simulink model "Feeder_1"  (Simulink 8.8)
settings: Solver=ode4  StartTime=0.0  StopTime=inf  FixedStep=Ts  RelTol=1e-3  EnableMultiTasking=on
PreLoadFcn:
  | Ts=125e-6;Core_Num = 0; np=1; nq=1; Vmin=.9;
PostLoadFcn:
  | Ts=125e-6;Core_Num = 0; np=1; nq=1; Vmin=.9;
InitFcn:
  | Ts=125e-6;Core_Num = 0; np=1; nq=1; Vmin=.9;
undefined symbols (not defined in the file or in its folder): another_event_name, DiscIntNeverNeededParam, I, j, Left, my_event_name, Right, type, V, X
libraries: powerlib x316, powerlib_meascontrol x227, simulink_extras x78, simulink x25, rtio_generic_c37_118 x22, ssn_lib x9, rtlab x6, powerlib_extras x3, artemis x1, rtio_opalrt_ml605ex1 x1, rtio_spectracom x1, rtio_generic_ethernet x1
(part 5 of 14)

== system Feeder_1/SS_PMU/Subsystem35 ==
  PMU in : Inport
  Bus Selector : BusSelector  OutputSignals=Measurements,FREQ,FROC
  Constant28 : Constant  Value=-1
  Constant29 : Constant  Value=-1
  Subsystem : Subsystem
  Phasors : Outport
  Analog : Outport  Port=2
  Ditigal : Outport  Port=3
  FREQ : Outport  Port=4
  FROC : Outport  Port=5
  wires:
  Subsystem/1(Out1) -> Bus Selector/1
  Bus Selector/1 -> Phasors/1  "<Measurements>"
  PMU in/1 -> Subsystem/1(In1)
  Constant28/1 -> Analog/1
  Constant29/1 -> Ditigal/1
  Bus Selector/2 -> FREQ/1  "<FREQ>"
  Bus Selector/3 -> FROC/1  "<FROC>"

== system Feeder_1/SS_PMU/Subsystem36 ==
  PMU in : Inport
  Bus Selector : BusSelector  OutputSignals=Measurements,FREQ,FROC
  Constant28 : Constant  Value=-1
  Constant29 : Constant  Value=-1
  Subsystem : Subsystem
  Phasors : Outport
  Analog : Outport  Port=2
  Ditigal : Outport  Port=3
  FREQ : Outport  Port=4
  FROC : Outport  Port=5
  wires:
  Subsystem/1(Out1) -> Bus Selector/1
  Bus Selector/1 -> Phasors/1  "<Measurements>"
  PMU in/1 -> Subsystem/1(In1)
  Constant28/1 -> Analog/1
  Constant29/1 -> Ditigal/1
  Bus Selector/2 -> FREQ/1  "<FREQ>"
  Bus Selector/3 -> FROC/1  "<FROC>"

== system Feeder_1/SS_PMU/Subsystem37 ==
  PMU in : Inport
  Bus Selector : BusSelector  OutputSignals=Measurements,FREQ,FROC
  Constant28 : Constant  Value=-1
  Constant29 : Constant  Value=-1
  Subsystem : Subsystem
  Phasors : Outport
  Analog : Outport  Port=2
  Ditigal : Outport  Port=3
  FREQ : Outport  Port=4
  FROC : Outport  Port=5
  wires:
  Subsystem/1(Out1) -> Bus Selector/1
  Bus Selector/1 -> Phasors/1  "<Measurements>"
  PMU in/1 -> Subsystem/1(In1)
  Constant28/1 -> Analog/1
  Constant29/1 -> Ditigal/1
  Bus Selector/2 -> FREQ/1  "<FREQ>"
  Bus Selector/3 -> FROC/1  "<FROC>"

== system Feeder_1/SS_PMU/Subsystem38 ==
  PMU in : Inport
  Bus Selector : BusSelector  OutputSignals=Measurements,FREQ,FROC
  Constant28 : Constant  Value=-1
  Constant29 : Constant  Value=-1
  Subsystem : Subsystem
  Phasors : Outport
  Analog : Outport  Port=2
  Ditigal : Outport  Port=3
  FREQ : Outport  Port=4
  FROC : Outport  Port=5
  wires:
  Subsystem/1(Out1) -> Bus Selector/1
  Bus Selector/1 -> Phasors/1  "<Measurements>"
  PMU in/1 -> Subsystem/1(In1)
  Constant28/1 -> Analog/1
  Constant29/1 -> Ditigal/1
  Bus Selector/2 -> FREQ/1  "<FREQ>"
  Bus Selector/3 -> FROC/1  "<FROC>"

== system Feeder_1/SS_PMU/Subsystem39 ==
  PMU in : Inport
  Bus Selector : BusSelector  OutputSignals=Measurements,FREQ,FROC
  Constant28 : Constant  Value=-1
  Constant29 : Constant  Value=-1
  Subsystem : Subsystem
  Phasors : Outport
  Analog : Outport  Port=2
  Ditigal : Outport  Port=3
  FREQ : Outport  Port=4
  FROC : Outport  Port=5
  wires:
  Subsystem/1(Out1) -> Bus Selector/1
  Bus Selector/1 -> Phasors/1  "<Measurements>"
  PMU in/1 -> Subsystem/1(In1)
  Constant28/1 -> Analog/1
  Constant29/1 -> Ditigal/1
  Bus Selector/2 -> FREQ/1  "<FREQ>"
  Bus Selector/3 -> FROC/1  "<FROC>"

== system Feeder_1/SS_PMU/Subsystem4 ==
  Measurements : Inport
  Demux7 : Demux  Outputs=6
  Demux8 : Demux  Outputs=6
  Mux5 : Mux  Inputs=12
  Subsystem : Subsystem
  Phasors : Outport
  Phasor_Freq : Outport  Port=2
  FROC : Outport  Port=3
  wires:
  Mux5/1 -> Phasors/1
  Demux7/4 -> [Phase_Va]
  Demux7/1 -> [Mag_Va]
  Demux7/2 -> [Mag_Vb]
  Demux7/3 -> [Mag_Vc]
  Subsystem/1(Phasors_Vabc) -> Demux7/1
  Demux7/6 -> [Phase_Vc]
  Demux7/5 -> [Phase_Vb]
  Subsystem/3(Phasor_Freq) -> Phasor_Freq/1
  Measurements/1 -> Subsystem/1(Measurements1)
  Subsystem/4(Phasor_DTFreq) -> FROC/1
  Demux8/2 -> [Mag_Ib]
  Demux8/4 -> [Phase_Ia]
  Demux8/5 -> [Phase_Ib]
  Subsystem/2(Phasors_Iabc) -> Demux8/1
  Demux8/3 -> [Mag_Ic]
  Demux8/1 -> [Mag_Ia]
  Demux8/6 -> [Phase_Ic]
  [Phase_Ic] -> Mux5/12
  [Mag_Ic] -> Mux5/11
  [Phase_Ib] -> Mux5/10
  [Mag_Ib] -> Mux5/9
  [Phase_Ia] -> Mux5/8
  [Mag_Ia] -> Mux5/7
  [Phase_Vc] -> Mux5/6
  [Mag_Vc] -> Mux5/5
  [Phase_Vb] -> Mux5/4
  [Mag_Vb] -> Mux5/3
  [Phase_Va] -> Mux5/2
  [Mag_Va] -> Mux5/1

== system Feeder_1/SS_PMU/Subsystem40 ==
  PMU in : Inport
  Bus Selector : BusSelector  OutputSignals=Measurements,FREQ,FROC
  Constant28 : Constant  Value=-1
  Constant29 : Constant  Value=-1
  Subsystem : Subsystem
  Phasors : Outport
  Analog : Outport  Port=2
  Ditigal : Outport  Port=3
  FREQ : Outport  Port=4
  FROC : Outport  Port=5
  wires:
  Subsystem/1(Out1) -> Bus Selector/1
  Bus Selector/1 -> Phasors/1  "<Measurements>"
  PMU in/1 -> Subsystem/1(In1)
  Constant28/1 -> Analog/1
  Constant29/1 -> Ditigal/1
  Bus Selector/2 -> FREQ/1  "<FREQ>"
  Bus Selector/3 -> FROC/1  "<FROC>"

== system Feeder_1/SS_PMU/Subsystem41 ==
  PMU in : Inport
  Bus Selector : BusSelector  OutputSignals=Measurements,FREQ,FROC
  Constant28 : Constant  Value=-1
  Constant29 : Constant  Value=-1
  Subsystem : Subsystem
  Phasors : Outport
  Analog : Outport  Port=2
  Ditigal : Outport  Port=3
  FREQ : Outport  Port=4
  FROC : Outport  Port=5
  wires:
  Subsystem/1(Out1) -> Bus Selector/1
  Bus Selector/1 -> Phasors/1  "<Measurements>"
  PMU in/1 -> Subsystem/1(In1)
  Constant28/1 -> Analog/1
  Constant29/1 -> Ditigal/1
  Bus Selector/2 -> FREQ/1  "<FREQ>"
  Bus Selector/3 -> FROC/1  "<FROC>"

== system Feeder_1/SS_PMU/Subsystem42 ==
  PMU in : Inport
  Bus Selector : BusSelector  OutputSignals=Measurements,FREQ,FROC
  Constant28 : Constant  Value=-1
  Constant29 : Constant  Value=-1
  Subsystem : Subsystem
  Phasors : Outport
  Analog : Outport  Port=2
  Ditigal : Outport  Port=3
  FREQ : Outport  Port=4
  FROC : Outport  Port=5
  wires:
  Subsystem/1(Out1) -> Bus Selector/1
  Bus Selector/1 -> Phasors/1  "<Measurements>"
  PMU in/1 -> Subsystem/1(In1)
  Constant28/1 -> Analog/1
  Constant29/1 -> Ditigal/1
  Bus Selector/2 -> FREQ/1  "<FREQ>"
  Bus Selector/3 -> FROC/1  "<FROC>"

== system Feeder_1/SS_PMU/Subsystem43 ==
  PMU in : Inport
  Bus Selector : BusSelector  OutputSignals=Measurements,FREQ,FROC
  Constant28 : Constant  Value=-1
  Constant29 : Constant  Value=-1
  Subsystem : Subsystem
  Phasors : Outport
  Analog : Outport  Port=2
  Ditigal : Outport  Port=3
  FREQ : Outport  Port=4
  FROC : Outport  Port=5
  wires:
  Subsystem/1(Out1) -> Bus Selector/1
  Bus Selector/1 -> Phasors/1  "<Measurements>"
  PMU in/1 -> Subsystem/1(In1)
  Constant28/1 -> Analog/1
  Constant29/1 -> Ditigal/1
  Bus Selector/2 -> FREQ/1  "<FREQ>"
  Bus Selector/3 -> FROC/1  "<FROC>"

== system Feeder_1/SS_PMU/Subsystem44 ==
  PMU in : Inport
  Bus Selector : BusSelector  OutputSignals=Measurements,FREQ,FROC
  Constant28 : Constant  Value=-1
  Constant29 : Constant  Value=-1
  Subsystem : Subsystem
  Phasors : Outport
  Analog : Outport  Port=2
  Ditigal : Outport  Port=3
  FREQ : Outport  Port=4
  FROC : Outport  Port=5
  wires:
  Subsystem/1(Out1) -> Bus Selector/1
  Bus Selector/1 -> Phasors/1  "<Measurements>"
  PMU in/1 -> Subsystem/1(In1)
  Constant28/1 -> Analog/1
  Constant29/1 -> Ditigal/1
  Bus Selector/2 -> FREQ/1  "<FREQ>"
  Bus Selector/3 -> FROC/1  "<FROC>"

== system Feeder_1/SS_PMU/Subsystem5 ==
  Measurements : Inport
  Demux7 : Demux  Outputs=6
  Demux8 : Demux  Outputs=6
  Mux5 : Mux  Inputs=12
  Subsystem : Subsystem
  Phasors : Outport
  Phasor_Freq : Outport  Port=2
  FROC : Outport  Port=3
  wires:
  Mux5/1 -> Phasors/1
  Demux7/4 -> [Phase_Va]
  Demux7/1 -> [Mag_Va]
  Demux7/2 -> [Mag_Vb]
  Demux7/3 -> [Mag_Vc]
  Subsystem/1(Phasors_Vabc) -> Demux7/1
  Demux7/6 -> [Phase_Vc]
  Demux7/5 -> [Phase_Vb]
  Subsystem/3(Phasor_Freq) -> Phasor_Freq/1
  Measurements/1 -> Subsystem/1(Measurements1)
  Subsystem/4(Phasor_DTFreq) -> FROC/1
  Demux8/2 -> [Mag_Ib]
  Demux8/4 -> [Phase_Ia]
  Demux8/5 -> [Phase_Ib]
  Subsystem/2(Phasors_Iabc) -> Demux8/1
  Demux8/3 -> [Mag_Ic]
  Demux8/1 -> [Mag_Ia]
  Demux8/6 -> [Phase_Ic]
  [Phase_Ic] -> Mux5/12
  [Mag_Ic] -> Mux5/11
  [Phase_Ib] -> Mux5/10
  [Mag_Ib] -> Mux5/9
  [Phase_Ia] -> Mux5/8
  [Mag_Ia] -> Mux5/7
  [Phase_Vc] -> Mux5/6
  [Mag_Vc] -> Mux5/5
  [Phase_Vb] -> Mux5/4
  [Mag_Vb] -> Mux5/3
  [Phase_Va] -> Mux5/2
  [Mag_Va] -> Mux5/1

== system Feeder_1/SS_PMU/Subsystem6 ==
  Measurements : Inport
  Demux7 : Demux  Outputs=6
  Demux8 : Demux  Outputs=6
  Mux5 : Mux  Inputs=12
  Subsystem : Subsystem
  Phasors : Outport
  Phasor_Freq : Outport  Port=2
  FROC : Outport  Port=3
  wires:
  Mux5/1 -> Phasors/1
  Demux7/4 -> [Phase_Va]
  Demux7/1 -> [Mag_Va]
  Demux7/2 -> [Mag_Vb]
  Demux7/3 -> [Mag_Vc]
  Subsystem/1(Phasors_Vabc) -> Demux7/1
  Demux7/6 -> [Phase_Vc]
  Demux7/5 -> [Phase_Vb]
  Subsystem/3(Phasor_Freq) -> Phasor_Freq/1
  Measurements/1 -> Subsystem/1(Measurements1)
  Subsystem/4(Phasor_DTFreq) -> FROC/1
  Demux8/2 -> [Mag_Ib]
  Demux8/4 -> [Phase_Ia]
  Demux8/5 -> [Phase_Ib]
  Subsystem/2(Phasors_Iabc) -> Demux8/1
  Demux8/3 -> [Mag_Ic]
  Demux8/1 -> [Mag_Ia]
  Demux8/6 -> [Phase_Ic]
  [Phase_Ic] -> Mux5/12
  [Mag_Ic] -> Mux5/11
  [Phase_Ib] -> Mux5/10
  [Mag_Ib] -> Mux5/9
  [Phase_Ia] -> Mux5/8
  [Mag_Ia] -> Mux5/7
  [Phase_Vc] -> Mux5/6
  [Mag_Vc] -> Mux5/5
  [Phase_Vb] -> Mux5/4
  [Mag_Vb] -> Mux5/3
  [Phase_Va] -> Mux5/2
  [Mag_Va] -> Mux5/1

== system Feeder_1/SS_PMU/Subsystem7 ==
  Measurements : Inport
  Demux7 : Demux  Outputs=6
  Demux8 : Demux  Outputs=6
  Mux5 : Mux  Inputs=12
  Subsystem : Subsystem
  Phasors : Outport
  Phasor_Freq : Outport  Port=2
  FROC : Outport  Port=3
  wires:
  Mux5/1 -> Phasors/1
  Demux7/4 -> [Phase_Va]
  Demux7/1 -> [Mag_Va]
  Demux7/2 -> [Mag_Vb]
  Demux7/3 -> [Mag_Vc]
  Subsystem/1(Phasors_Vabc) -> Demux7/1
  Demux7/6 -> [Phase_Vc]
  Demux7/5 -> [Phase_Vb]
  Subsystem/3(Phasor_Freq) -> Phasor_Freq/1
  Measurements/1 -> Subsystem/1(Measurements1)
  Subsystem/4(Phasor_DTFreq) -> FROC/1
  Demux8/2 -> [Mag_Ib]
  Demux8/4 -> [Phase_Ia]
  Demux8/5 -> [Phase_Ib]
  Subsystem/2(Phasors_Iabc) -> Demux8/1
  Demux8/3 -> [Mag_Ic]
  Demux8/1 -> [Mag_Ia]
  Demux8/6 -> [Phase_Ic]
  [Phase_Ic] -> Mux5/12
  [Mag_Ic] -> Mux5/11
  [Phase_Ib] -> Mux5/10
  [Mag_Ib] -> Mux5/9
  [Phase_Ia] -> Mux5/8
  [Mag_Ia] -> Mux5/7
  [Phase_Vc] -> Mux5/6
  [Mag_Vc] -> Mux5/5
  [Phase_Vb] -> Mux5/4
  [Mag_Vb] -> Mux5/3
  [Phase_Va] -> Mux5/2
  [Mag_Va] -> Mux5/1

== system Feeder_1/SS_PMU/Subsystem8 ==
  Measurements : Inport
  Demux7 : Demux  Outputs=6
  Demux8 : Demux  Outputs=6
  Mux5 : Mux  Inputs=12
  Subsystem : Subsystem
  Phasors : Outport
  Phasor_Freq : Outport  Port=2
  FROC : Outport  Port=3
  wires:
  Mux5/1 -> Phasors/1
  Demux7/4 -> [Phase_Va]
  Demux7/1 -> [Mag_Va]
  Demux7/2 -> [Mag_Vb]
  Demux7/3 -> [Mag_Vc]
  Subsystem/1(Phasors_Vabc) -> Demux7/1
  Demux7/6 -> [Phase_Vc]
  Demux7/5 -> [Phase_Vb]
  Subsystem/3(Phasor_Freq) -> Phasor_Freq/1
  Measurements/1 -> Subsystem/1(Measurements1)
  Subsystem/4(Phasor_DTFreq) -> FROC/1
  Demux8/2 -> [Mag_Ib]
  Demux8/4 -> [Phase_Ia]
  Demux8/5 -> [Phase_Ib]
  Subsystem/2(Phasors_Iabc) -> Demux8/1
  Demux8/3 -> [Mag_Ic]
  Demux8/1 -> [Mag_Ia]
  Demux8/6 -> [Phase_Ic]
  [Phase_Ic] -> Mux5/12
  [Mag_Ic] -> Mux5/11
  [Phase_Ib] -> Mux5/10
  [Mag_Ib] -> Mux5/9
  [Phase_Ia] -> Mux5/8
  [Mag_Ia] -> Mux5/7
  [Phase_Vc] -> Mux5/6
  [Mag_Vc] -> Mux5/5
  [Phase_Vb] -> Mux5/4
  [Mag_Vb] -> Mux5/3
  [Phase_Va] -> Mux5/2
  [Mag_Va] -> Mux5/1

== system Feeder_1/SS_PMU/Subsystem9 ==
  Measurements : Inport
  Demux7 : Demux  Outputs=6
  Demux8 : Demux  Outputs=6
  Mux5 : Mux  Inputs=12
  Subsystem : Subsystem
  Phasors : Outport
  Phasor_Freq : Outport  Port=2
  FROC : Outport  Port=3
  wires:
  Mux5/1 -> Phasors/1
  Demux7/4 -> [Phase_Va]
  Demux7/1 -> [Mag_Va]
  Demux7/2 -> [Mag_Vb]
  Demux7/3 -> [Mag_Vc]
  Subsystem/1(Phasors_Vabc) -> Demux7/1
  Demux7/6 -> [Phase_Vc]
  Demux7/5 -> [Phase_Vb]
  Subsystem/3(Phasor_Freq) -> Phasor_Freq/1
  Measurements/1 -> Subsystem/1(Measurements1)
  Subsystem/4(Phasor_DTFreq) -> FROC/1
  Demux8/2 -> [Mag_Ib]
  Demux8/4 -> [Phase_Ia]
  Demux8/5 -> [Phase_Ib]
  Subsystem/2(Phasors_Iabc) -> Demux8/1
  Demux8/3 -> [Mag_Ic]
  Demux8/1 -> [Mag_Ia]
  Demux8/6 -> [Phase_Ic]
  [Phase_Ic] -> Mux5/12
  [Mag_Ic] -> Mux5/11
  [Phase_Ib] -> Mux5/10
  [Mag_Ib] -> Mux5/9
  [Phase_Ia] -> Mux5/8
  [Mag_Ia] -> Mux5/7
  [Phase_Vc] -> Mux5/6
  [Mag_Vc] -> Mux5/5
  [Phase_Vb] -> Mux5/4
  [Mag_Vb] -> Mux5/3
  [Phase_Va] -> Mux5/2
  [Mag_Va] -> Mux5/1

== system Feeder_1/SM_NG/Dynamic Load BCDC2/Single-Phase Dynamic Load1 ==
  P : Inport
  Q : Inport  Port=2
  Active : Gain  Gain=900000
  Active1 : Gain  Gain=400000
  Controlled Current Source : powerlib/Electrical Sources/Controlled Current Source  Initialize=on  Source_Type=AC  Amplitude=0  Phase=0  Frequency=0  Measurements=None
  Gain : Gain  Gain=-1
  Mux8 : Mux  Inputs=2
  Voltage Measurement1 : powerlib/Measurements/Voltage Measurement  PhasorSimulation=off  OutputType=Complex  PSBequivalent=0
  model : Subsystem
  a : PMIOPort  Tag=PMCPort  Port=1  Side=Left
  b : PMIOPort  Tag=PMCPort  Port=2  Side=Left
  wires:
  Mux8/1 -> model/2(PQ)
  Voltage Measurement1/1 -> model/1(v)
  model/1(i) -> Gain/1
  Gain/1 -> Controlled Current Source/1
  Active/1 -> Mux8/1
  Active1/1 -> Mux8/2
  P/1 -> Active/1
  Q/1 -> Active1/1
  connections:
  Voltage Measurement1/LConn1 -- a/RConn1 -- Controlled Current Source/RConn1
  Voltage Measurement1/LConn2 -- b/RConn1 -- Controlled Current Source/LConn1

== system Feeder_1/SM_NG/Dynamic Load BCDC2/Single-Phase Dynamic Load2 ==
  P : Inport
  Q : Inport  Port=2
  Active : Gain  Gain=500000
  Active1 : Gain  Gain=400000
  Controlled Current Source : powerlib/Electrical Sources/Controlled Current Source  Initialize=on  Source_Type=AC  Amplitude=0  Phase=0  Frequency=0  Measurements=None
  Gain : Gain  Gain=-1
  Mux8 : Mux  Inputs=2
  Voltage Measurement1 : powerlib/Measurements/Voltage Measurement  PhasorSimulation=off  OutputType=Complex  PSBequivalent=0
  model : Subsystem
  a : PMIOPort  Tag=PMCPort  Port=1  Side=Left
  b : PMIOPort  Tag=PMCPort  Port=2  Side=Left
  wires:
  Mux8/1 -> model/2(PQ)
  Voltage Measurement1/1 -> model/1(v)
  model/1(i) -> Gain/1
  Gain/1 -> Controlled Current Source/1
  Active/1 -> Mux8/1
  Active1/1 -> Mux8/2
  P/1 -> Active/1
  Q/1 -> Active1/1
  connections:
  Voltage Measurement1/LConn1 -- a/RConn1 -- Controlled Current Source/RConn1
  Voltage Measurement1/LConn2 -- b/RConn1 -- Controlled Current Source/LConn1

== system Feeder_1/SM_NG/Dynamic Load BCDC2/Single-Phase Dynamic Load9 ==
  P : Inport
  Q : Inport  Port=2
  Active : Gain  Gain=400000
  Active1 : Gain  Gain=300000
  Controlled Current Source : powerlib/Electrical Sources/Controlled Current Source  Initialize=on  Source_Type=AC  Amplitude=0  Phase=0  Frequency=0  Measurements=None
  Gain : Gain  Gain=-1
  Mux8 : Mux  Inputs=2
  Voltage Measurement1 : powerlib/Measurements/Voltage Measurement  PhasorSimulation=off  OutputType=Complex  PSBequivalent=0
  model : Subsystem
  a : PMIOPort  Tag=PMCPort  Port=1  Side=Left
  b : PMIOPort  Tag=PMCPort  Port=2  Side=Left
  wires:
  Voltage Measurement1/1 -> model/1(v)
  model/1(i) -> Gain/1
  Gain/1 -> Controlled Current Source/1
  Active/1 -> Mux8/1
  Mux8/1 -> model/2(PQ)
  Active1/1 -> Mux8/2
  P/1 -> Active/1
  Q/1 -> Active1/1
  connections:
  Voltage Measurement1/LConn1 -- a/RConn1 -- Controlled Current Source/RConn1
  Voltage Measurement1/LConn2 -- b/RConn1 -- Controlled Current Source/LConn1

== system Feeder_1/SM_NG/Dynamic Load BCDC3/Single-Phase Dynamic Load1 ==
  P : Inport
  Q : Inport  Port=2
  Active : Gain  Gain=300000
  Active1 : Gain  Gain=100000
  Controlled Current Source : powerlib/Electrical Sources/Controlled Current Source  Initialize=on  Source_Type=AC  Amplitude=0  Phase=0  Frequency=0  Measurements=None
  Gain : Gain  Gain=-1
  Mux8 : Mux  Inputs=2
  Voltage Measurement1 : powerlib/Measurements/Voltage Measurement  PhasorSimulation=off  OutputType=Complex  PSBequivalent=0
  model : Subsystem
  a : PMIOPort  Tag=PMCPort  Port=1  Side=Left
  b : PMIOPort  Tag=PMCPort  Port=2  Side=Left
  wires:
  Mux8/1 -> model/2(PQ)
  Voltage Measurement1/1 -> model/1(v)
  model/1(i) -> Gain/1
  Gain/1 -> Controlled Current Source/1
  Active/1 -> Mux8/1
  Active1/1 -> Mux8/2
  P/1 -> Active/1
  Q/1 -> Active1/1
  connections:
  Voltage Measurement1/LConn1 -- a/RConn1 -- Controlled Current Source/RConn1
  Voltage Measurement1/LConn2 -- b/RConn1 -- Controlled Current Source/LConn1

== system Feeder_1/SM_NG/Dynamic Load BCDC3/Single-Phase Dynamic Load2 ==
  P : Inport
  Q : Inport  Port=2
  Active : Gain  Gain=100000
  Active1 : Gain  Gain=100000
  Controlled Current Source : powerlib/Electrical Sources/Controlled Current Source  Initialize=on  Source_Type=AC  Amplitude=0  Phase=0  Frequency=0  Measurements=None
  Gain : Gain  Gain=-1
  Mux8 : Mux  Inputs=2
  Voltage Measurement1 : powerlib/Measurements/Voltage Measurement  PhasorSimulation=off  OutputType=Complex  PSBequivalent=0
  model : Subsystem
  a : PMIOPort  Tag=PMCPort  Port=1  Side=Left
  b : PMIOPort  Tag=PMCPort  Port=2  Side=Left
  wires:
  Mux8/1 -> model/2(PQ)
  Voltage Measurement1/1 -> model/1(v)
  model/1(i) -> Gain/1
  Gain/1 -> Controlled Current Source/1
  Active/1 -> Mux8/1
  Active1/1 -> Mux8/2
  P/1 -> Active/1
  Q/1 -> Active1/1
  connections:
  Voltage Measurement1/LConn1 -- a/RConn1 -- Controlled Current Source/RConn1
  Voltage Measurement1/LConn2 -- b/RConn1 -- Controlled Current Source/LConn1

== system Feeder_1/SM_NG/Dynamic Load BCDC3/Single-Phase Dynamic Load9 ==
  P : Inport
  Q : Inport  Port=2
  Active : Gain  Gain=300000
  Active1 : Gain  Gain=200000
  Controlled Current Source : powerlib/Electrical Sources/Controlled Current Source  Initialize=on  Source_Type=AC  Amplitude=0  Phase=0  Frequency=0  Measurements=None
  Gain : Gain  Gain=-1
  Mux8 : Mux  Inputs=2
  Voltage Measurement1 : powerlib/Measurements/Voltage Measurement  PhasorSimulation=off  OutputType=Complex  PSBequivalent=0
  model : Subsystem
  a : PMIOPort  Tag=PMCPort  Port=1  Side=Left
  b : PMIOPort  Tag=PMCPort  Port=2  Side=Left
  wires:
  Voltage Measurement1/1 -> model/1(v)
  model/1(i) -> Gain/1
  Gain/1 -> Controlled Current Source/1
  Active/1 -> Mux8/1
  Mux8/1 -> model/2(PQ)
  Active1/1 -> Mux8/2
  P/1 -> Active/1
  Q/1 -> Active1/1
  connections:
  Voltage Measurement1/LConn1 -- a/RConn1 -- Controlled Current Source/RConn1
  Voltage Measurement1/LConn2 -- b/RConn1 -- Controlled Current Source/LConn1

== system Feeder_1/SM_NG/Dynamic Load BCDC4/Single-Phase Dynamic Load1 ==
  P : Inport
  Q : Inport  Port=2
  Active : Gain  Gain=300000
  Active1 : Gain  Gain=100000
  Controlled Current Source : powerlib/Electrical Sources/Controlled Current Source  Initialize=on  Source_Type=AC  Amplitude=0  Phase=0  Frequency=0  Measurements=None
  Gain : Gain  Gain=-1
  Mux8 : Mux  Inputs=2
  Voltage Measurement1 : powerlib/Measurements/Voltage Measurement  PhasorSimulation=off  OutputType=Complex  PSBequivalent=0
  model : Subsystem
  a : PMIOPort  Tag=PMCPort  Port=1  Side=Left
  b : PMIOPort  Tag=PMCPort  Port=2  Side=Left
  wires:
  Mux8/1 -> model/2(PQ)
  Voltage Measurement1/1 -> model/1(v)
  model/1(i) -> Gain/1
  Gain/1 -> Controlled Current Source/1
  Active/1 -> Mux8/1
  Active1/1 -> Mux8/2
  P/1 -> Active/1
  Q/1 -> Active1/1
  connections:
  Voltage Measurement1/LConn1 -- a/RConn1 -- Controlled Current Source/RConn1
  Voltage Measurement1/LConn2 -- b/RConn1 -- Controlled Current Source/LConn1

== system Feeder_1/SM_NG/Dynamic Load BCDC4/Single-Phase Dynamic Load2 ==
  P : Inport
  Q : Inport  Port=2
  Active : Gain  Gain=100000
  Active1 : Gain  Gain=100000
  Controlled Current Source : powerlib/Electrical Sources/Controlled Current Source  Initialize=on  Source_Type=AC  Amplitude=0  Phase=0  Frequency=0  Measurements=None
  Gain : Gain  Gain=-1
  Mux8 : Mux  Inputs=2
  Voltage Measurement1 : powerlib/Measurements/Voltage Measurement  PhasorSimulation=off  OutputType=Complex  PSBequivalent=0
  model : Subsystem
  a : PMIOPort  Tag=PMCPort  Port=1  Side=Left
  b : PMIOPort  Tag=PMCPort  Port=2  Side=Left
  wires:
  Mux8/1 -> model/2(PQ)
  Voltage Measurement1/1 -> model/1(v)
  model/1(i) -> Gain/1
  Gain/1 -> Controlled Current Source/1
  Active/1 -> Mux8/1
  Active1/1 -> Mux8/2
  P/1 -> Active/1
  Q/1 -> Active1/1
  connections:
  Voltage Measurement1/LConn1 -- a/RConn1 -- Controlled Current Source/RConn1
  Voltage Measurement1/LConn2 -- b/RConn1 -- Controlled Current Source/LConn1

== system Feeder_1/SM_NG/Dynamic Load BCDC4/Single-Phase Dynamic Load9 ==
  P : Inport
  Q : Inport  Port=2
  Active : Gain  Gain=300000
  Active1 : Gain  Gain=200000
  Controlled Current Source : powerlib/Electrical Sources/Controlled Current Source  Initialize=on  Source_Type=AC  Amplitude=0  Phase=0  Frequency=0  Measurements=None
  Gain : Gain  Gain=-1
  Mux8 : Mux  Inputs=2
  Voltage Measurement1 : powerlib/Measurements/Voltage Measurement  PhasorSimulation=off  OutputType=Complex  PSBequivalent=0
  model : Subsystem
  a : PMIOPort  Tag=PMCPort  Port=1  Side=Left
  b : PMIOPort  Tag=PMCPort  Port=2  Side=Left
  wires:
  Voltage Measurement1/1 -> model/1(v)
  model/1(i) -> Gain/1
  Gain/1 -> Controlled Current Source/1
  Active/1 -> Mux8/1
  Mux8/1 -> model/2(PQ)
  Active1/1 -> Mux8/2
  P/1 -> Active/1
  Q/1 -> Active1/1
  connections:
  Voltage Measurement1/LConn1 -- a/RConn1 -- Controlled Current Source/RConn1
  Voltage Measurement1/LConn2 -- b/RConn1 -- Controlled Current Source/LConn1

== system Feeder_1/SM_NG/Single-Phase Dynamic Load30/model ==
  v : Inport
  PQ : Inport  Port=2
  -Q : Gain  SaturateOnIntegerOverflow=on  OutDataTypeStr=Inherit: Same as input  ParamDataTypeStr=Inherit: Same as input
  Break  Alg. Loop1 : Subsystem
  Complex to Magnitude-Angle : ComplexToMagnitudeAngle
  Complex to Real-Imag1 : ComplexToRealImag
  Constant : Constant
  Demux : Demux  Outputs=2
  Divide : Product  Inputs=**
  Gain : Gain  Gain=1.0114
  IC1 : InitialCondition
  IC2 : InitialCondition
  Magnitude-Angle to Complex : MagnitudeAngleToComplex
  PLL : Subsystem  mask{freq=fnom}
      mask prompts: freq "Initial frequency (Hz)"
  Positive Sequence  current : Subsystem
  RMS1 : powerlib_meascontrol/Measurements/RMS  TrueRMS=on  Freq=fnom  RMSInit=1  Ts=0
  Real-Imag to Complex : RealImagToComplex
  Real-Imag to Complex1 : RealImagToComplex
  Sum : Sum
  Transfer Fcn1 : TransferFcn  Numerator=[1 290.1]  Denominator=[1 298.8]
  Trigonometric Function1 : Trigonometry
  V> pu : Gain  Gain=1/Vbase/sqrt(3)  SaturateOnIntegerOverflow=on  OutDataTypeStr=Inherit: Same as input  ParamDataTypeStr=Inherit: Same as input
  V> pu1 : Gain  Gain=sqrt(2)  SaturateOnIntegerOverflow=on  OutDataTypeStr=Inherit: Same as input  ParamDataTypeStr=Inherit: Same as input
  i : Outport
  wires:
  V> pu/1 -> PLL/1(v (pu)), V> pu1/1
  Real-Imag to Complex/1 -> Positive Sequence  current/1(V1(pu))
  PQ/1 -> Demux/1
  Demux/1 -> Real-Imag to Complex1/1
  Demux/2 -> -Q/1
  Real-Imag to Complex1/1 -> Positive Sequence  current/2(S_ext)
  Complex to Real-Imag1/1 -> Real-Imag to Complex/1
  Complex to Real-Imag1/2 -> Real-Imag to Complex/2
  Magnitude-Angle to Complex/1 -> Complex to Real-Imag1/1
  Constant/1 -> PLL/2(freq (pu))
  PLL/1(alpha (rad)) -> Magnitude-Angle to Complex/2
  Complex to Magnitude-Angle/2 -> Sum/2
  PLL/2(wt) -> Sum/1
  Sum/1 -> Trigonometric Function1/1
  Trigonometric Function1/1 -> Divide/2
  Complex to Magnitude-Angle/1 -> Divide/1
  RMS1/1 -> IC1/1
  V> pu1/1 -> RMS1/1
  v/1 -> IC2/1
  Positive Sequence  current/1(I1(A)) -> Break  Alg. Loop1/1(In)
  Break  Alg. Loop1/1(Out) -> Complex to Magnitude-Angle/1
  IC1/1 -> Magnitude-Angle to Complex/1
  IC2/1 -> V> pu/1
  Transfer Fcn1/1 -> Gain/1
  Gain/1 -> i/1
  Divide/1 -> Transfer Fcn1/1
  -Q/1 -> Real-Imag to Complex1/2

== system Feeder_1/SM_NG/Single-Phase Dynamic Load32/model ==
  v : Inport
  PQ : Inport  Port=2
  -Q : Gain  SaturateOnIntegerOverflow=on  OutDataTypeStr=Inherit: Same as input  ParamDataTypeStr=Inherit: Same as input
  Break  Alg. Loop1 : Subsystem
  Complex to Magnitude-Angle : ComplexToMagnitudeAngle
  Complex to Real-Imag1 : ComplexToRealImag
  Constant : Constant
  Demux : Demux  Outputs=2
  Divide : Product  Inputs=**
  Gain : Gain  Gain=1.0114
  IC1 : InitialCondition
  IC2 : InitialCondition
  Magnitude-Angle to Complex : MagnitudeAngleToComplex
  PLL : Subsystem  mask{freq=fnom}
      mask prompts: freq "Initial frequency (Hz)"
  Positive Sequence  current : Subsystem
  RMS1 : powerlib_meascontrol/Measurements/RMS  TrueRMS=on  Freq=fnom  RMSInit=1  Ts=0
  Real-Imag to Complex : RealImagToComplex
  Real-Imag to Complex1 : RealImagToComplex
  Sum : Sum
  Transfer Fcn1 : TransferFcn  Numerator=[1 290.1]  Denominator=[1 298.8]
  Trigonometric Function1 : Trigonometry
  V> pu : Gain  Gain=1/Vbase/sqrt(3)  SaturateOnIntegerOverflow=on  OutDataTypeStr=Inherit: Same as input  ParamDataTypeStr=Inherit: Same as input
  V> pu1 : Gain  Gain=sqrt(2)  SaturateOnIntegerOverflow=on  OutDataTypeStr=Inherit: Same as input  ParamDataTypeStr=Inherit: Same as input
  i : Outport
  wires:
  V> pu/1 -> PLL/1(v (pu)), V> pu1/1
  Real-Imag to Complex/1 -> Positive Sequence  current/1(V1(pu))
  PQ/1 -> Demux/1
  Demux/1 -> Real-Imag to Complex1/1
  Demux/2 -> -Q/1
  Real-Imag to Complex1/1 -> Positive Sequence  current/2(S_ext)
  Complex to Real-Imag1/1 -> Real-Imag to Complex/1
  Complex to Real-Imag1/2 -> Real-Imag to Complex/2
  Magnitude-Angle to Complex/1 -> Complex to Real-Imag1/1
  Constant/1 -> PLL/2(freq (pu))
  PLL/1(alpha (rad)) -> Magnitude-Angle to Complex/2
  Complex to Magnitude-Angle/2 -> Sum/2
  PLL/2(wt) -> Sum/1
  Sum/1 -> Trigonometric Function1/1
  Trigonometric Function1/1 -> Divide/2
  Complex to Magnitude-Angle/1 -> Divide/1
  RMS1/1 -> IC1/1
  V> pu1/1 -> RMS1/1
  v/1 -> IC2/1
  Positive Sequence  current/1(I1(A)) -> Break  Alg. Loop1/1(In)
  Break  Alg. Loop1/1(Out) -> Complex to Magnitude-Angle/1
  IC1/1 -> Magnitude-Angle to Complex/1
  IC2/1 -> V> pu/1
  Transfer Fcn1/1 -> Gain/1
  Gain/1 -> i/1
  Divide/1 -> Transfer Fcn1/1
  -Q/1 -> Real-Imag to Complex1/2

== system Feeder_1/SM_NG/Single-Phase Dynamic Load33/model ==
  v : Inport
  PQ : Inport  Port=2
  -Q : Gain  SaturateOnIntegerOverflow=on  OutDataTypeStr=Inherit: Same as input  ParamDataTypeStr=Inherit: Same as input
  Break  Alg. Loop1 : Subsystem
  Complex to Magnitude-Angle : ComplexToMagnitudeAngle
  Complex to Real-Imag1 : ComplexToRealImag
  Constant : Constant
  Demux : Demux  Outputs=2
  Divide : Product  Inputs=**
  Gain : Gain  Gain=1.0114
  IC1 : InitialCondition
  IC2 : InitialCondition
  Magnitude-Angle to Complex : MagnitudeAngleToComplex
  PLL : Subsystem  mask{freq=fnom}
      mask prompts: freq "Initial frequency (Hz)"
  Positive Sequence  current : Subsystem
  RMS1 : powerlib_meascontrol/Measurements/RMS  TrueRMS=on  Freq=fnom  RMSInit=1  Ts=0
  Real-Imag to Complex : RealImagToComplex
  Real-Imag to Complex1 : RealImagToComplex
  Sum : Sum
  Transfer Fcn1 : TransferFcn  Numerator=[1 290.1]  Denominator=[1 298.8]
  Trigonometric Function1 : Trigonometry
  V> pu : Gain  Gain=1/Vbase/sqrt(3)  SaturateOnIntegerOverflow=on  OutDataTypeStr=Inherit: Same as input  ParamDataTypeStr=Inherit: Same as input
  V> pu1 : Gain  Gain=sqrt(2)  SaturateOnIntegerOverflow=on  OutDataTypeStr=Inherit: Same as input  ParamDataTypeStr=Inherit: Same as input
  i : Outport
  wires:
  V> pu/1 -> PLL/1(v (pu)), V> pu1/1
  Real-Imag to Complex/1 -> Positive Sequence  current/1(V1(pu))
  PQ/1 -> Demux/1
  Demux/1 -> Real-Imag to Complex1/1
  Demux/2 -> -Q/1
  Real-Imag to Complex1/1 -> Positive Sequence  current/2(S_ext)
  Complex to Real-Imag1/1 -> Real-Imag to Complex/1
  Complex to Real-Imag1/2 -> Real-Imag to Complex/2
  Magnitude-Angle to Complex/1 -> Complex to Real-Imag1/1
  Constant/1 -> PLL/2(freq (pu))
  PLL/1(alpha (rad)) -> Magnitude-Angle to Complex/2
  Complex to Magnitude-Angle/2 -> Sum/2
  PLL/2(wt) -> Sum/1
  Sum/1 -> Trigonometric Function1/1
  Trigonometric Function1/1 -> Divide/2
  Complex to Magnitude-Angle/1 -> Divide/1
  RMS1/1 -> IC1/1
  V> pu1/1 -> RMS1/1
  v/1 -> IC2/1
  Positive Sequence  current/1(I1(A)) -> Break  Alg. Loop1/1(In)
  Break  Alg. Loop1/1(Out) -> Complex to Magnitude-Angle/1
  IC1/1 -> Magnitude-Angle to Complex/1
  IC2/1 -> V> pu/1
  Transfer Fcn1/1 -> Gain/1
  Gain/1 -> i/1
  Divide/1 -> Transfer Fcn1/1
  -Q/1 -> Real-Imag to Complex1/2

== system Feeder_1/SM_NG/Single-Phase Dynamic Load34/model ==
  v : Inport
  PQ : Inport  Port=2
  -Q : Gain  SaturateOnIntegerOverflow=on  OutDataTypeStr=Inherit: Same as input  ParamDataTypeStr=Inherit: Same as input
  Break  Alg. Loop1 : Subsystem
  Complex to Magnitude-Angle : ComplexToMagnitudeAngle
  Complex to Real-Imag1 : ComplexToRealImag
  Constant : Constant
  Demux : Demux  Outputs=2
  Divide : Product  Inputs=**
  Gain : Gain  Gain=1.0114
  IC1 : InitialCondition
  IC2 : InitialCondition
  Magnitude-Angle to Complex : MagnitudeAngleToComplex
  PLL : Subsystem  mask{freq=fnom}
      mask prompts: freq "Initial frequency (Hz)"
  Positive Sequence  current : Subsystem
  RMS1 : powerlib_meascontrol/Measurements/RMS  TrueRMS=on  Freq=fnom  RMSInit=1  Ts=0
  Real-Imag to Complex : RealImagToComplex
  Real-Imag to Complex1 : RealImagToComplex
  Sum : Sum
  Transfer Fcn1 : TransferFcn  Numerator=[1 290.1]  Denominator=[1 298.8]
  Trigonometric Function1 : Trigonometry
  V> pu : Gain  Gain=1/Vbase/sqrt(3)  SaturateOnIntegerOverflow=on  OutDataTypeStr=Inherit: Same as input  ParamDataTypeStr=Inherit: Same as input
  V> pu1 : Gain  Gain=sqrt(2)  SaturateOnIntegerOverflow=on  OutDataTypeStr=Inherit: Same as input  ParamDataTypeStr=Inherit: Same as input
  i : Outport
  wires:
  V> pu/1 -> PLL/1(v (pu)), V> pu1/1
  Real-Imag to Complex/1 -> Positive Sequence  current/1(V1(pu))
  PQ/1 -> Demux/1
  Demux/1 -> Real-Imag to Complex1/1
  Demux/2 -> -Q/1
  Real-Imag to Complex1/1 -> Positive Sequence  current/2(S_ext)
  Complex to Real-Imag1/1 -> Real-Imag to Complex/1
  Complex to Real-Imag1/2 -> Real-Imag to Complex/2
  Magnitude-Angle to Complex/1 -> Complex to Real-Imag1/1
  Constant/1 -> PLL/2(freq (pu))
  PLL/1(alpha (rad)) -> Magnitude-Angle to Complex/2
  Complex to Magnitude-Angle/2 -> Sum/2
  PLL/2(wt) -> Sum/1
  Sum/1 -> Trigonometric Function1/1
  Trigonometric Function1/1 -> Divide/2
  Complex to Magnitude-Angle/1 -> Divide/1
  RMS1/1 -> IC1/1
  V> pu1/1 -> RMS1/1
  v/1 -> IC2/1
  Positive Sequence  current/1(I1(A)) -> Break  Alg. Loop1/1(In)
  Break  Alg. Loop1/1(Out) -> Complex to Magnitude-Angle/1
  IC1/1 -> Magnitude-Angle to Complex/1
  IC2/1 -> V> pu/1
  Transfer Fcn1/1 -> Gain/1
  Gain/1 -> i/1
  Divide/1 -> Transfer Fcn1/1
  -Q/1 -> Real-Imag to Complex1/2

== system Feeder_1/SM_NG/Single-Phase Dynamic Load35/model ==
  v : Inport
  PQ : Inport  Port=2
  -Q : Gain  SaturateOnIntegerOverflow=on  OutDataTypeStr=Inherit: Same as input  ParamDataTypeStr=Inherit: Same as input
  Break  Alg. Loop : Subsystem
  Complex to Magnitude-Angle : ComplexToMagnitudeAngle
  Complex to Real-Imag1 : ComplexToRealImag
  Constant : Constant
  Demux : Demux  Outputs=2
  Divide : Product  Inputs=**
  Gain : Gain  Gain=1.0114
  IC1 : InitialCondition
  IC2 : InitialCondition
  Magnitude-Angle to Complex : MagnitudeAngleToComplex
  PLL : Subsystem  mask{freq=fnom}
      mask prompts: freq "Initial frequency (Hz)"
  Positive Sequence  current : Subsystem
  RMS1 : powerlib_meascontrol/Measurements/RMS  TrueRMS=on  Freq=fnom  RMSInit=1  Ts=0
  Real-Imag to Complex : RealImagToComplex
  Real-Imag to Complex1 : RealImagToComplex
  Sum : Sum
  Transfer Fcn1 : TransferFcn  Numerator=[1 290.1]  Denominator=[1 298.8]
  Trigonometric Function1 : Trigonometry
  V> pu : Gain  Gain=1/Vbase/sqrt(3)  SaturateOnIntegerOverflow=on  OutDataTypeStr=Inherit: Same as input  ParamDataTypeStr=Inherit: Same as input
  V> pu1 : Gain  Gain=sqrt(2)  SaturateOnIntegerOverflow=on  OutDataTypeStr=Inherit: Same as input  ParamDataTypeStr=Inherit: Same as input
  i : Outport
  wires:
  V> pu/1 -> PLL/1(v (pu)), V> pu1/1
  Real-Imag to Complex/1 -> Positive Sequence  current/1(V1(pu))
  Positive Sequence  current/1(I1(A)) -> Break  Alg. Loop/1(In)
  PQ/1 -> Demux/1
  Demux/1 -> Real-Imag to Complex1/1
  Demux/2 -> -Q/1
  Real-Imag to Complex1/1 -> Positive Sequence  current/2(S_ext)
  v/1 -> IC2/1
  Complex to Real-Imag1/1 -> Real-Imag to Complex/1
  Complex to Real-Imag1/2 -> Real-Imag to Complex/2
  Magnitude-Angle to Complex/1 -> Complex to Real-Imag1/1
  Constant/1 -> PLL/2(freq (pu))
  PLL/1(alpha (rad)) -> Magnitude-Angle to Complex/2
  Complex to Magnitude-Angle/2 -> Sum/2
  PLL/2(wt) -> Sum/1
  Sum/1 -> Trigonometric Function1/1
  Trigonometric Function1/1 -> Divide/2
  Complex to Magnitude-Angle/1 -> Divide/1
  Break  Alg. Loop/1(Out) -> Complex to Magnitude-Angle/1
  RMS1/1 -> IC1/1
  IC1/1 -> Magnitude-Angle to Complex/1
  V> pu1/1 -> RMS1/1
  IC2/1 -> V> pu/1
  -Q/1 -> Real-Imag to Complex1/2
  Transfer Fcn1/1 -> Gain/1
  Divide/1 -> Transfer Fcn1/1
  Gain/1 -> i/1

== system Feeder_1/SM_NG/Single-Phase Dynamic Load36/model ==
  v : Inport
  PQ : Inport  Port=2
  -Q : Gain  SaturateOnIntegerOverflow=on  OutDataTypeStr=Inherit: Same as input  ParamDataTypeStr=Inherit: Same as input
  Break  Alg. Loop1 : Subsystem
  Complex to Magnitude-Angle : ComplexToMagnitudeAngle
  Complex to Real-Imag1 : ComplexToRealImag
  Constant : Constant
  Demux : Demux  Outputs=2
  Divide : Product  Inputs=**
  Gain : Gain  Gain=1.0114
  IC1 : InitialCondition
  IC2 : InitialCondition
  Magnitude-Angle to Complex : MagnitudeAngleToComplex
  PLL : Subsystem  mask{freq=fnom}
      mask prompts: freq "Initial frequency (Hz)"
  Positive Sequence  current : Subsystem
  RMS1 : powerlib_meascontrol/Measurements/RMS  TrueRMS=on  Freq=fnom  RMSInit=1  Ts=0
  Real-Imag to Complex : RealImagToComplex
  Real-Imag to Complex1 : RealImagToComplex
  Sum : Sum
  Transfer Fcn1 : TransferFcn  Numerator=[1 290.1]  Denominator=[1 298.8]
  Trigonometric Function1 : Trigonometry
  V> pu : Gain  Gain=1/Vbase/sqrt(3)  SaturateOnIntegerOverflow=on  OutDataTypeStr=Inherit: Same as input  ParamDataTypeStr=Inherit: Same as input
  V> pu1 : Gain  Gain=sqrt(2)  SaturateOnIntegerOverflow=on  OutDataTypeStr=Inherit: Same as input  ParamDataTypeStr=Inherit: Same as input
  i : Outport
  wires:
  V> pu/1 -> PLL/1(v (pu)), V> pu1/1
  Real-Imag to Complex/1 -> Positive Sequence  current/1(V1(pu))
  PQ/1 -> Demux/1
  Demux/1 -> Real-Imag to Complex1/1
  Demux/2 -> -Q/1
  Real-Imag to Complex1/1 -> Positive Sequence  current/2(S_ext)
  Complex to Real-Imag1/1 -> Real-Imag to Complex/1
  Complex to Real-Imag1/2 -> Real-Imag to Complex/2
  Magnitude-Angle to Complex/1 -> Complex to Real-Imag1/1
  Constant/1 -> PLL/2(freq (pu))
  PLL/1(alpha (rad)) -> Magnitude-Angle to Complex/2
  Complex to Magnitude-Angle/2 -> Sum/2
  PLL/2(wt) -> Sum/1
  Sum/1 -> Trigonometric Function1/1
  Trigonometric Function1/1 -> Divide/2
  Complex to Magnitude-Angle/1 -> Divide/1
  RMS1/1 -> IC1/1
  V> pu1/1 -> RMS1/1
  v/1 -> IC2/1
  Positive Sequence  current/1(I1(A)) -> Break  Alg. Loop1/1(In)
  Break  Alg. Loop1/1(Out) -> Complex to Magnitude-Angle/1
  IC1/1 -> Magnitude-Angle to Complex/1
  IC2/1 -> V> pu/1
  Transfer Fcn1/1 -> Gain/1
  Gain/1 -> i/1
  Divide/1 -> Transfer Fcn1/1
  -Q/1 -> Real-Imag to Complex1/2

== system Feeder_1/SM_NG/Single-Phase Dynamic Load37/model ==
  v : Inport
  PQ : Inport  Port=2
  -Q : Gain  SaturateOnIntegerOverflow=on  OutDataTypeStr=Inherit: Same as input  ParamDataTypeStr=Inherit: Same as input
  Break  Alg. Loop1 : Subsystem
  Complex to Magnitude-Angle : ComplexToMagnitudeAngle
  Complex to Real-Imag1 : ComplexToRealImag
  Constant : Constant
  Demux : Demux  Outputs=2
  Divide : Product  Inputs=**
  Gain : Gain  Gain=1.0114
  IC1 : InitialCondition
  IC2 : InitialCondition
  Magnitude-Angle to Complex : MagnitudeAngleToComplex
  PLL : Subsystem  mask{freq=fnom}
      mask prompts: freq "Initial frequency (Hz)"
  Positive Sequence  current : Subsystem
  RMS1 : powerlib_meascontrol/Measurements/RMS  TrueRMS=on  Freq=fnom  RMSInit=1  Ts=0
  Real-Imag to Complex : RealImagToComplex
  Real-Imag to Complex1 : RealImagToComplex
  Sum : Sum
  Transfer Fcn1 : TransferFcn  Numerator=[1 290.1]  Denominator=[1 298.8]
  Trigonometric Function1 : Trigonometry
  V> pu : Gain  Gain=1/Vbase/sqrt(3)  SaturateOnIntegerOverflow=on  OutDataTypeStr=Inherit: Same as input  ParamDataTypeStr=Inherit: Same as input
  V> pu1 : Gain  Gain=sqrt(2)  SaturateOnIntegerOverflow=on  OutDataTypeStr=Inherit: Same as input  ParamDataTypeStr=Inherit: Same as input
  i : Outport
  wires:
  V> pu/1 -> PLL/1(v (pu)), V> pu1/1
  Real-Imag to Complex/1 -> Positive Sequence  current/1(V1(pu))
  PQ/1 -> Demux/1
  Demux/1 -> Real-Imag to Complex1/1
  Demux/2 -> -Q/1
  Real-Imag to Complex1/1 -> Positive Sequence  current/2(S_ext)
  Complex to Real-Imag1/1 -> Real-Imag to Complex/1
  Complex to Real-Imag1/2 -> Real-Imag to Complex/2
  Magnitude-Angle to Complex/1 -> Complex to Real-Imag1/1
  Constant/1 -> PLL/2(freq (pu))
  PLL/1(alpha (rad)) -> Magnitude-Angle to Complex/2
  Complex to Magnitude-Angle/2 -> Sum/2
  PLL/2(wt) -> Sum/1
  Sum/1 -> Trigonometric Function1/1
  Trigonometric Function1/1 -> Divide/2
  Complex to Magnitude-Angle/1 -> Divide/1
  RMS1/1 -> IC1/1
  V> pu1/1 -> RMS1/1
  v/1 -> IC2/1
  Positive Sequence  current/1(I1(A)) -> Break  Alg. Loop1/1(In)
  Break  Alg. Loop1/1(Out) -> Complex to Magnitude-Angle/1
  IC1/1 -> Magnitude-Angle to Complex/1
  IC2/1 -> V> pu/1
  Transfer Fcn1/1 -> Gain/1
  Gain/1 -> i/1
  Divide/1 -> Transfer Fcn1/1
  -Q/1 -> Real-Imag to Complex1/2

== system Feeder_1/SM_NG/Single-Phase Dynamic Load38/model ==
  v : Inport
  PQ : Inport  Port=2
  -Q : Gain  SaturateOnIntegerOverflow=on  OutDataTypeStr=Inherit: Same as input  ParamDataTypeStr=Inherit: Same as input
  Break  Alg. Loop1 : Subsystem
  Complex to Magnitude-Angle : ComplexToMagnitudeAngle
  Complex to Real-Imag1 : ComplexToRealImag
  Constant : Constant
  Demux : Demux  Outputs=2
  Divide : Product  Inputs=**
  Gain : Gain  Gain=1.0114
  IC1 : InitialCondition
  IC2 : InitialCondition
  Magnitude-Angle to Complex : MagnitudeAngleToComplex
  PLL : Subsystem  mask{freq=fnom}
      mask prompts: freq "Initial frequency (Hz)"
  Positive Sequence  current : Subsystem
  RMS1 : powerlib_meascontrol/Measurements/RMS  TrueRMS=on  Freq=fnom  RMSInit=1  Ts=0
  Real-Imag to Complex : RealImagToComplex
  Real-Imag to Complex1 : RealImagToComplex
  Sum : Sum
  Transfer Fcn1 : TransferFcn  Numerator=[1 290.1]  Denominator=[1 298.8]
  Trigonometric Function1 : Trigonometry
  V> pu : Gain  Gain=1/Vbase/sqrt(3)  SaturateOnIntegerOverflow=on  OutDataTypeStr=Inherit: Same as input  ParamDataTypeStr=Inherit: Same as input
  V> pu1 : Gain  Gain=sqrt(2)  SaturateOnIntegerOverflow=on  OutDataTypeStr=Inherit: Same as input  ParamDataTypeStr=Inherit: Same as input
  i : Outport
  wires:
  V> pu/1 -> PLL/1(v (pu)), V> pu1/1
  Real-Imag to Complex/1 -> Positive Sequence  current/1(V1(pu))
  PQ/1 -> Demux/1
  Demux/1 -> Real-Imag to Complex1/1
  Demux/2 -> -Q/1
  Real-Imag to Complex1/1 -> Positive Sequence  current/2(S_ext)
  Complex to Real-Imag1/1 -> Real-Imag to Complex/1
  Complex to Real-Imag1/2 -> Real-Imag to Complex/2
  Magnitude-Angle to Complex/1 -> Complex to Real-Imag1/1
  Constant/1 -> PLL/2(freq (pu))
  PLL/1(alpha (rad)) -> Magnitude-Angle to Complex/2
  Complex to Magnitude-Angle/2 -> Sum/2
  PLL/2(wt) -> Sum/1
  Sum/1 -> Trigonometric Function1/1
  Trigonometric Function1/1 -> Divide/2
  Complex to Magnitude-Angle/1 -> Divide/1
  RMS1/1 -> IC1/1
  V> pu1/1 -> RMS1/1
  v/1 -> IC2/1
  Positive Sequence  current/1(I1(A)) -> Break  Alg. Loop1/1(In)
  Break  Alg. Loop1/1(Out) -> Complex to Magnitude-Angle/1
  IC1/1 -> Magnitude-Angle to Complex/1
  IC2/1 -> V> pu/1
  Transfer Fcn1/1 -> Gain/1
  Gain/1 -> i/1
  Divide/1 -> Transfer Fcn1/1
  -Q/1 -> Real-Imag to Complex1/2

== system Feeder_1/SM_NG/Single-Phase Dynamic Load39/model ==
  v : Inport
  PQ : Inport  Port=2
  -Q : Gain  SaturateOnIntegerOverflow=on  OutDataTypeStr=Inherit: Same as input  ParamDataTypeStr=Inherit: Same as input
  Break  Alg. Loop1 : Subsystem
  Complex to Magnitude-Angle : ComplexToMagnitudeAngle
  Complex to Real-Imag1 : ComplexToRealImag
  Constant : Constant
  Demux : Demux  Outputs=2
  Divide : Product  Inputs=**
  Gain : Gain  Gain=1.0114
  IC1 : InitialCondition
  IC2 : InitialCondition
  Magnitude-Angle to Complex : MagnitudeAngleToComplex
  PLL : Subsystem  mask{freq=fnom}
      mask prompts: freq "Initial frequency (Hz)"
  Positive Sequence  current : Subsystem
  RMS1 : powerlib_meascontrol/Measurements/RMS  TrueRMS=on  Freq=fnom  RMSInit=1  Ts=0
  Real-Imag to Complex : RealImagToComplex
  Real-Imag to Complex1 : RealImagToComplex
  Sum : Sum
  Transfer Fcn1 : TransferFcn  Numerator=[1 290.1]  Denominator=[1 298.8]
  Trigonometric Function1 : Trigonometry
  V> pu : Gain  Gain=1/Vbase/sqrt(3)  SaturateOnIntegerOverflow=on  OutDataTypeStr=Inherit: Same as input  ParamDataTypeStr=Inherit: Same as input
  V> pu1 : Gain  Gain=sqrt(2)  SaturateOnIntegerOverflow=on  OutDataTypeStr=Inherit: Same as input  ParamDataTypeStr=Inherit: Same as input
  i : Outport
  wires:
  V> pu/1 -> PLL/1(v (pu)), V> pu1/1
  Real-Imag to Complex/1 -> Positive Sequence  current/1(V1(pu))
  PQ/1 -> Demux/1
  Demux/1 -> Real-Imag to Complex1/1
  Demux/2 -> -Q/1
  Real-Imag to Complex1/1 -> Positive Sequence  current/2(S_ext)
  Complex to Real-Imag1/1 -> Real-Imag to Complex/1
  Complex to Real-Imag1/2 -> Real-Imag to Complex/2
  Magnitude-Angle to Complex/1 -> Complex to Real-Imag1/1
  Constant/1 -> PLL/2(freq (pu))
  PLL/1(alpha (rad)) -> Magnitude-Angle to Complex/2
  Complex to Magnitude-Angle/2 -> Sum/2
  PLL/2(wt) -> Sum/1
  Sum/1 -> Trigonometric Function1/1
  Trigonometric Function1/1 -> Divide/2
  Complex to Magnitude-Angle/1 -> Divide/1
  RMS1/1 -> IC1/1
  V> pu1/1 -> RMS1/1
  v/1 -> IC2/1
  Positive Sequence  current/1(I1(A)) -> Break  Alg. Loop1/1(In)
  Break  Alg. Loop1/1(Out) -> Complex to Magnitude-Angle/1
  IC1/1 -> Magnitude-Angle to Complex/1
  IC2/1 -> V> pu/1
  Transfer Fcn1/1 -> Gain/1
  Gain/1 -> i/1
  Divide/1 -> Transfer Fcn1/1
  -Q/1 -> Real-Imag to Complex1/2

== system Feeder_1/SM_NG/Single-Phase Dynamic Load40/model ==
  v : Inport
  PQ : Inport  Port=2
  -Q : Gain  SaturateOnIntegerOverflow=on  OutDataTypeStr=Inherit: Same as input  ParamDataTypeStr=Inherit: Same as input
  Break  Alg. Loop1 : Subsystem
  Complex to Magnitude-Angle : ComplexToMagnitudeAngle
  Complex to Real-Imag1 : ComplexToRealImag
  Constant : Constant
  Demux : Demux  Outputs=2
  Divide : Product  Inputs=**
  Gain : Gain  Gain=1.01
  IC1 : InitialCondition
  IC2 : InitialCondition
  Magnitude-Angle to Complex : MagnitudeAngleToComplex
  PLL : Subsystem  mask{freq=fnom}
      mask prompts: freq "Initial frequency (Hz)"
  Positive Sequence  current : Subsystem
  RMS1 : powerlib_meascontrol/Measurements/RMS  TrueRMS=on  Freq=fnom  RMSInit=1  Ts=0
  Real-Imag to Complex : RealImagToComplex
  Real-Imag to Complex1 : RealImagToComplex
  Sum : Sum
  Transfer Fcn1 : TransferFcn  Numerator=[1 290.1]  Denominator=[1 298.8]
  Trigonometric Function1 : Trigonometry
  V> pu : Gain  Gain=1/Vbase/sqrt(3)  SaturateOnIntegerOverflow=on  OutDataTypeStr=Inherit: Same as input  ParamDataTypeStr=Inherit: Same as input
  V> pu1 : Gain  Gain=sqrt(2)  SaturateOnIntegerOverflow=on  OutDataTypeStr=Inherit: Same as input  ParamDataTypeStr=Inherit: Same as input
  i : Outport
  wires:
  V> pu/1 -> PLL/1(v (pu)), V> pu1/1
  Real-Imag to Complex/1 -> Positive Sequence  current/1(V1(pu))
  PQ/1 -> Demux/1
  Demux/1 -> Real-Imag to Complex1/1
  Demux/2 -> -Q/1
  Real-Imag to Complex1/1 -> Positive Sequence  current/2(S_ext)
  Complex to Real-Imag1/1 -> Real-Imag to Complex/1
  Complex to Real-Imag1/2 -> Real-Imag to Complex/2
  Magnitude-Angle to Complex/1 -> Complex to Real-Imag1/1
  Constant/1 -> PLL/2(freq (pu))
  PLL/1(alpha (rad)) -> Magnitude-Angle to Complex/2
  Complex to Magnitude-Angle/2 -> Sum/2
  PLL/2(wt) -> Sum/1
  Sum/1 -> Trigonometric Function1/1
  Trigonometric Function1/1 -> Divide/2
  Complex to Magnitude-Angle/1 -> Divide/1
  RMS1/1 -> IC1/1
  V> pu1/1 -> RMS1/1
  v/1 -> IC2/1
  Positive Sequence  current/1(I1(A)) -> Break  Alg. Loop1/1(In)
  Break  Alg. Loop1/1(Out) -> Complex to Magnitude-Angle/1
  IC1/1 -> Magnitude-Angle to Complex/1
  IC2/1 -> V> pu/1
  Transfer Fcn1/1 -> Gain/1
  Gain/1 -> i/1
  Divide/1 -> Transfer Fcn1/1
  -Q/1 -> Real-Imag to Complex1/2

== system Feeder_1/SM_NG/Single-Phase Dynamic Load41/model ==
  v : Inport
  PQ : Inport  Port=2
  -Q : Gain  SaturateOnIntegerOverflow=on  OutDataTypeStr=Inherit: Same as input  ParamDataTypeStr=Inherit: Same as input
  Break  Alg. Loop1 : Subsystem
  Complex to Magnitude-Angle : ComplexToMagnitudeAngle
  Complex to Real-Imag1 : ComplexToRealImag
  Constant : Constant
  Demux : Demux  Outputs=2
  Divide : Product  Inputs=**
  Gain : Gain  Gain=1.0114
  IC1 : InitialCondition
  IC2 : InitialCondition
  Magnitude-Angle to Complex : MagnitudeAngleToComplex
  PLL : Subsystem  mask{freq=fnom}
      mask prompts: freq "Initial frequency (Hz)"
  Positive Sequence  current : Subsystem
  RMS1 : powerlib_meascontrol/Measurements/RMS  TrueRMS=on  Freq=fnom  RMSInit=1  Ts=0
  Real-Imag to Complex : RealImagToComplex
  Real-Imag to Complex1 : RealImagToComplex
  Sum : Sum
  Transfer Fcn1 : TransferFcn  Numerator=[1 290.1]  Denominator=[1 298.8]
  Trigonometric Function1 : Trigonometry
  V> pu : Gain  Gain=1/Vbase/sqrt(3)  SaturateOnIntegerOverflow=on  OutDataTypeStr=Inherit: Same as input  ParamDataTypeStr=Inherit: Same as input
  V> pu1 : Gain  Gain=sqrt(2)  SaturateOnIntegerOverflow=on  OutDataTypeStr=Inherit: Same as input  ParamDataTypeStr=Inherit: Same as input
  i : Outport
  wires:
  V> pu/1 -> PLL/1(v (pu)), V> pu1/1
  Real-Imag to Complex/1 -> Positive Sequence  current/1(V1(pu))
  PQ/1 -> Demux/1
  Demux/1 -> Real-Imag to Complex1/1
  Demux/2 -> -Q/1
  Real-Imag to Complex1/1 -> Positive Sequence  current/2(S_ext)
  Complex to Real-Imag1/1 -> Real-Imag to Complex/1
  Complex to Real-Imag1/2 -> Real-Imag to Complex/2
  Magnitude-Angle to Complex/1 -> Complex to Real-Imag1/1
  Constant/1 -> PLL/2(freq (pu))
  PLL/1(alpha (rad)) -> Magnitude-Angle to Complex/2
  Complex to Magnitude-Angle/2 -> Sum/2
  PLL/2(wt) -> Sum/1
  Sum/1 -> Trigonometric Function1/1
  Trigonometric Function1/1 -> Divide/2
  Complex to Magnitude-Angle/1 -> Divide/1
  RMS1/1 -> IC1/1
  V> pu1/1 -> RMS1/1
  v/1 -> IC2/1
  Positive Sequence  current/1(I1(A)) -> Break  Alg. Loop1/1(In)
  Break  Alg. Loop1/1(Out) -> Complex to Magnitude-Angle/1
  IC1/1 -> Magnitude-Angle to Complex/1
  IC2/1 -> V> pu/1
  Transfer Fcn1/1 -> Gain/1
  Gain/1 -> i/1
  Divide/1 -> Transfer Fcn1/1
  -Q/1 -> Real-Imag to Complex1/2

== system Feeder_1/SM_NG/Single-Phase Dynamic Load42/model ==
  v : Inport
  PQ : Inport  Port=2
  -Q : Gain  SaturateOnIntegerOverflow=on  OutDataTypeStr=Inherit: Same as input  ParamDataTypeStr=Inherit: Same as input
  Break  Alg. Loop1 : Subsystem
  Complex to Magnitude-Angle : ComplexToMagnitudeAngle
  Complex to Real-Imag1 : ComplexToRealImag
  Constant : Constant
  Demux : Demux  Outputs=2
  Divide : Product  Inputs=**
  Gain : Gain  Gain=1.0114
  IC1 : InitialCondition
  IC2 : InitialCondition
  Magnitude-Angle to Complex : MagnitudeAngleToComplex
  PLL : Subsystem  mask{freq=fnom}
      mask prompts: freq "Initial frequency (Hz)"
  Positive Sequence  current : Subsystem
  RMS1 : powerlib_meascontrol/Measurements/RMS  TrueRMS=on  Freq=fnom  RMSInit=1  Ts=0
  Real-Imag to Complex : RealImagToComplex
  Real-Imag to Complex1 : RealImagToComplex
  Sum : Sum
  Transfer Fcn1 : TransferFcn  Numerator=[1 290.1]  Denominator=[1 298.8]
  Trigonometric Function1 : Trigonometry
  V> pu : Gain  Gain=1/Vbase/sqrt(3)  SaturateOnIntegerOverflow=on  OutDataTypeStr=Inherit: Same as input  ParamDataTypeStr=Inherit: Same as input
  V> pu1 : Gain  Gain=sqrt(2)  SaturateOnIntegerOverflow=on  OutDataTypeStr=Inherit: Same as input  ParamDataTypeStr=Inherit: Same as input
  i : Outport
  wires:
  V> pu/1 -> PLL/1(v (pu)), V> pu1/1
  Real-Imag to Complex/1 -> Positive Sequence  current/1(V1(pu))
  PQ/1 -> Demux/1
  Demux/1 -> Real-Imag to Complex1/1
  Demux/2 -> -Q/1
  Real-Imag to Complex1/1 -> Positive Sequence  current/2(S_ext)
  Complex to Real-Imag1/1 -> Real-Imag to Complex/1
  Complex to Real-Imag1/2 -> Real-Imag to Complex/2
  Magnitude-Angle to Complex/1 -> Complex to Real-Imag1/1
  Constant/1 -> PLL/2(freq (pu))
  PLL/1(alpha (rad)) -> Magnitude-Angle to Complex/2
  Complex to Magnitude-Angle/2 -> Sum/2
  PLL/2(wt) -> Sum/1
  Sum/1 -> Trigonometric Function1/1
  Trigonometric Function1/1 -> Divide/2
  Complex to Magnitude-Angle/1 -> Divide/1
  RMS1/1 -> IC1/1
  V> pu1/1 -> RMS1/1
  v/1 -> IC2/1
  Positive Sequence  current/1(I1(A)) -> Break  Alg. Loop1/1(In)
  Break  Alg. Loop1/1(Out) -> Complex to Magnitude-Angle/1
  IC1/1 -> Magnitude-Angle to Complex/1
  IC2/1 -> V> pu/1
  Transfer Fcn1/1 -> Gain/1
  Gain/1 -> i/1
  Divide/1 -> Transfer Fcn1/1
  -Q/1 -> Real-Imag to Complex1/2
